simulink model "COSTEP_Exergy"  (R2024b)
settings: Solver=FixedStepAuto  StartTime=0.0  StopTime=25  FixedStep=1/3600  RelTol=1e-3
model workspace (MAT data in the model file):
  AD : Simulink.Parameter (value not decoded)
  AG : Simulink.Parameter (value not decoded)
  AH : Simulink.Parameter (value not decoded)
  AV : Simulink.Parameter (value not decoded)
  AVP : Simulink.Parameter (value not decoded)
  BCHL : Simulink.Parameter (value not decoded)
  BCHV : Simulink.Parameter (value not decoded)
  BD : Simulink.Parameter (value not decoded)
  BDIST : Simulink.Parameter (value not decoded)
  BG : Simulink.Parameter (value not decoded)
  BH : Simulink.Parameter (value not decoded)
  BVP : Simulink.Parameter (value not decoded)
  CD : Simulink.Parameter (value not decoded)
  CDIST : Simulink.Parameter (value not decoded)
  CG : Simulink.Parameter (value not decoded)
  CH : Simulink.Parameter (value not decoded)
  CVP : Simulink.Parameter (value not decoded)
  DDIST : Simulink.Parameter (value not decoded)
  DIST_CONST : Simulink.Parameter (value not decoded)
  ISV : Simulink.Parameter (value not decoded)
  TLAST : Simulink.Parameter (value not decoded)
  TNEXT : Simulink.Parameter (value not decoded)
  XMW : Simulink.Parameter (value not decoded)
  XNS : Simulink.Parameter (value not decoded)
  XNS2 : Simulink.Parameter (value not decoded)
  XNS3 : Simulink.Parameter (value not decoded)
  XNSADD : Simulink.Parameter (value not decoded)
  XNSE : Simulink.Parameter (value not decoded)
symbols that are objects in the model workspace (value not decoded): AD, AG, AH, AV, AVP, BD, BG, BH, BVP, CD, CG, CH, CVP, XMW, XNS, XNS2, XNS3, XNSE
undefined symbols (not defined in the file or in its folder): magnitude, msgbox, SETPT, XMEAS, XMV
libraries: mylib x403, dspindex x31
(part 8 of 13)

== system COSTEP_Exergy/Stripper/Holdup of Components in Stripper/Holsup of Liquid Components in Stripper ==
  YY(19:26) : Inport
  Bus Creator : BusCreator  Inputs=8
  Bus Selector : BusSelector  OutputSignals=YY(19),YY(20),YY(21),YY(22),YY(23),YY(24),YY(25),YY(26)
  UCLC(1) Holdup of Component A (Liquid) in Stripper lb-mol : Gain
  UCLC(2) Holdup of Component B (Liquid) in Stripper lb-mol : Gain
  UCLC(3) Holdup of Component C (Liquid) in Stripper lb-mol : Gain
  UCLC(4) Holdup of Component D (Liquid) in Stripper lb-mol : Gain
  UCLC(5) Holdup of Component E (Liquid) in Stripper lb-mol : Gain
  UCLC(6) Holdup of Component F (Liquid) in Stripper lb-mol : Gain
  UCLC(7) Holdup of Component G (Liquid) in Stripper lb-mol : Gain
  UCLC(8) Holdup of Component H (Liquid) in Stripper lb-mol : Gain
  UCLC : Outport  VectorParamsAs1DForOutWhenUnconnected=off
  wires:
  UCLC(8) Holdup of Component H (Liquid) in Stripper lb-mol/1 -> Bus Creator/8
  UCLC(2) Holdup of Component B (Liquid) in Stripper lb-mol/1 -> Bus Creator/2
  UCLC(1) Holdup of Component A (Liquid) in Stripper lb-mol/1 -> Bus Creator/1
  Bus Creator/1 -> UCLC/1
  UCLC(5) Holdup of Component E (Liquid) in Stripper lb-mol/1 -> Bus Creator/5
  UCLC(7) Holdup of Component G (Liquid) in Stripper lb-mol/1 -> Bus Creator/7
  UCLC(4) Holdup of Component D (Liquid) in Stripper lb-mol/1 -> Bus Creator/4
  UCLC(6) Holdup of Component F (Liquid) in Stripper lb-mol/1 -> Bus Creator/6
  UCLC(3) Holdup of Component C (Liquid) in Stripper lb-mol/1 -> Bus Creator/3
  YY(19:26)/1 -> Bus Selector/1
  Bus Selector/1 -> UCLC(1) Holdup of Component A (Liquid) in Stripper lb-mol/1  "<YY(19)>"
  Bus Selector/2 -> UCLC(2) Holdup of Component B (Liquid) in Stripper lb-mol/1  "<YY(20)>"
  Bus Selector/3 -> UCLC(3) Holdup of Component C (Liquid) in Stripper lb-mol/1  "<YY(21)>"
  Bus Selector/4 -> UCLC(4) Holdup of Component D (Liquid) in Stripper lb-mol/1  "<YY(22)>"
  Bus Selector/5 -> UCLC(5) Holdup of Component E (Liquid) in Stripper lb-mol/1  "<YY(23)>"
  Bus Selector/6 -> UCLC(6) Holdup of Component F (Liquid) in Stripper lb-mol/1  "<YY(24)>"
  Bus Selector/7 -> UCLC(7) Holdup of Component G (Liquid) in Stripper lb-mol/1  "<YY(25)>"
  Bus Selector/8 -> UCLC(8) Holdup of Component H (Liquid) in Stripper lb-mol/1  "<YY(26)>"

== system COSTEP_Exergy/Stripper/Holdup of Components in Stripper/Liquid Component Fraction in Stripper ==
  UTLC : Inport
  UCLC : Inport  Port=2
  Bus Selector : BusSelector  OutputSignals=signal1,signal2,signal3,signal4,signal5,signal6,signal7,signal8
  Mux : Mux  Inputs=8
  XLC(1) : Product  Inputs=*/
  XLC(2) : Product  Inputs=*/
  XLC(3) : Product  Inputs=*/
  XLC(4) : Product  Inputs=*/
  XLC(5) : Product  Inputs=*/
  XLC(6) : Product  Inputs=*/
  XLC(7) : Product  Inputs=*/
  XLC(8) : Product  Inputs=*/
  XLC : Outport  VectorParamsAs1DForOutWhenUnconnected=off
  wires:
  XLC(3)/1 -> Mux/3  "XLC(3)"
  Bus Selector/2 -> XLC(2)/1  "<signal2>"
  Bus Selector/7 -> XLC(7)/1  "<signal7>"
  XLC(5)/1 -> Mux/5  "XLC(5)"
  XLC(7)/1 -> Mux/7  "XLC(7)"
  Bus Selector/3 -> XLC(3)/1  "<signal3>"
  UTLC/1 -> XLC(8)/2, XLC(7)/2, XLC(6)/2, XLC(5)/2, XLC(4)/2, XLC(3)/2, XLC(2)/2, XLC(1)/2
  Bus Selector/6 -> XLC(6)/1  "<signal6>"
  Bus Selector/5 -> XLC(5)/1  "<signal5>"
  XLC(2)/1 -> Mux/2  "XLC(2)"
  XLC(6)/1 -> Mux/6  "XLC(6)"
  Bus Selector/4 -> XLC(4)/1  "<signal4>"
  XLC(1)/1 -> Mux/1  "XLC(1)"
  XLC(8)/1 -> Mux/8  "XLC(8)"
  UCLC/1 -> Bus Selector/1
  XLC(4)/1 -> Mux/4  "XLC(4)"
  Mux/1 -> XLC/1
  Bus Selector/1 -> XLC(1)/1  "<signal1>"
  Bus Selector/8 -> XLC(8)/1  "<signal8>"

== system COSTEP_Exergy/Stripper/Holdup of Components in Stripper/YP(19) ==
  FCM(1,12) : Inport
  FCM(1,13) : Inport  Port=2
  " " : Sum  Inputs=+-
  Constant : Constant  Value=19
  Initial state variable : mylib/Initial state variable
  Integration : mylib/Integration  SystemSampleTime=-1  VariantActivationTime=update diagram  AllowFlexibleInterface=on  Latency=0  AutoFrameSizeCalculation=off
  YY(19) : Outport  VectorParamsAs1DForOutWhenUnconnected=off
  wires:
  Initial state variable/1 -> Integration/2
  FCM(1,13)/1 -> " "/2
  FCM(1,12)/1 -> " "/1
  " "/1 -> Integration/1
  Integration/1 -> YY(19)/1
  Constant/1 -> Initial state variable/1

== system COSTEP_Exergy/Stripper/Holdup of Components in Stripper/YP(20) ==
  FCM(2,12) : Inport
  FCM(2,13) : Inport  Port=2
  " " : Sum  Inputs=+-
  Constant : Constant  Value=20
  Initial state variable : mylib/Initial state variable
  Integration : mylib/Integration  SystemSampleTime=-1  VariantActivationTime=update diagram  AllowFlexibleInterface=on  Latency=0  AutoFrameSizeCalculation=off
  YY(20) : Outport  VectorParamsAs1DForOutWhenUnconnected=off
  wires:
  Integration/1 -> YY(20)/1
  FCM(2,12)/1 -> " "/1
  FCM(2,13)/1 -> " "/2
  Initial state variable/1 -> Integration/2
  " "/1 -> Integration/1
  Constant/1 -> Initial state variable/1

== system COSTEP_Exergy/Stripper/Holdup of Components in Stripper/YP(21) ==
  FCM(3,12) : Inport
  FCM(3,13) : Inport  Port=2
  " " : Sum  Inputs=+-
  Constant : Constant  Value=21
  Initial state variable : mylib/Initial state variable
  Integration : mylib/Integration  SystemSampleTime=-1  VariantActivationTime=update diagram  AllowFlexibleInterface=on  Latency=0  AutoFrameSizeCalculation=off
  YY(21) : Outport  VectorParamsAs1DForOutWhenUnconnected=off
  wires:
  Integration/1 -> YY(21)/1
  FCM(3,12)/1 -> " "/1
  FCM(3,13)/1 -> " "/2
  " "/1 -> Integration/1
  Initial state variable/1 -> Integration/2
  Constant/1 -> Initial state variable/1

== system COSTEP_Exergy/Stripper/Holdup of Components in Stripper/YP(22) ==
  FCM(4,12) : Inport
  FCM(4,13) : Inport  Port=2
  " " : Sum  Inputs=+-
  Constant : Constant  Value=22
  Initial state variable : mylib/Initial state variable
  Integration : mylib/Integration  SystemSampleTime=-1  VariantActivationTime=update diagram  AllowFlexibleInterface=on  Latency=0  AutoFrameSizeCalculation=off
  "YY(22)  " : Outport  VectorParamsAs1DForOutWhenUnconnected=off
  wires:
  Integration/1 -> "YY(22)  "/1
  FCM(4,12)/1 -> " "/1
  FCM(4,13)/1 -> " "/2
  " "/1 -> Integration/1
  Initial state variable/1 -> Integration/2
  Constant/1 -> Initial state variable/1

== system COSTEP_Exergy/Stripper/Holdup of Components in Stripper/YP(23) ==
  FCM(5,12) : Inport
  FCM(5,13) : Inport  Port=2
  " " : Sum  Inputs=+-
  Constant : Constant  Value=23
  Initial state variable : mylib/Initial state variable
  Integration : mylib/Integration  SystemSampleTime=-1  VariantActivationTime=update diagram  AllowFlexibleInterface=on  Latency=0  AutoFrameSizeCalculation=off
  "YY(23)  " : Outport  VectorParamsAs1DForOutWhenUnconnected=off
  wires:
  Integration/1 -> "YY(23)  "/1
  FCM(5,12)/1 -> " "/1
  FCM(5,13)/1 -> " "/2
  " "/1 -> Integration/1
  Initial state variable/1 -> Integration/2
  Constant/1 -> Initial state variable/1

== system COSTEP_Exergy/Stripper/Holdup of Components in Stripper/YP(24) ==
  FCM(6,12) : Inport
  FCM(6,13) : Inport  Port=2
  " " : Sum  Inputs=+-
  Constant : Constant  Value=24
  Initial state variable : mylib/Initial state variable
  Integration : mylib/Integration  SystemSampleTime=-1  VariantActivationTime=update diagram  AllowFlexibleInterface=on  Latency=0  AutoFrameSizeCalculation=off
  "YY(24)  " : Outport  VectorParamsAs1DForOutWhenUnconnected=off
  wires:
  Integration/1 -> "YY(24)  "/1
  FCM(6,12)/1 -> " "/1
  FCM(6,13)/1 -> " "/2
  " "/1 -> Integration/1
  Initial state variable/1 -> Integration/2
  Constant/1 -> Initial state variable/1

== system COSTEP_Exergy/Stripper/Holdup of Components in Stripper/YP(25) ==
  FCM(7,12) : Inport
  FCM(7,13) : Inport  Port=2
  " " : Sum  Inputs=+-
  Constant : Constant  Value=25
  Initial state variable : mylib/Initial state variable
  Integration : mylib/Integration  SystemSampleTime=-1  VariantActivationTime=update diagram  AllowFlexibleInterface=on  Latency=0  AutoFrameSizeCalculation=off
  "YY(25)  " : Outport  VectorParamsAs1DForOutWhenUnconnected=off
  wires:
  Integration/1 -> "YY(25)  "/1
  FCM(7,12)/1 -> " "/1
  FCM(7,13)/1 -> " "/2
  " "/1 -> Integration/1
  Initial state variable/1 -> Integration/2
  Constant/1 -> Initial state variable/1

== system COSTEP_Exergy/Stripper/Holdup of Components in Stripper/YP(26) ==
  FCM(8,12) : Inport
  FCM(8,13) : Inport  Port=2
  " " : Sum  Inputs=+-
  Constant : Constant  Value=26
  Initial state variable : mylib/Initial state variable
  Integration : mylib/Integration  SystemSampleTime=-1  VariantActivationTime=update diagram  AllowFlexibleInterface=on  Latency=0  AutoFrameSizeCalculation=off
  "YY(26)   " : Outport  VectorParamsAs1DForOutWhenUnconnected=off
  wires:
  Integration/1 -> "YY(26)   "/1
  FCM(8,12)/1 -> " "/1
  FCM(8,13)/1 -> " "/2
  " "/1 -> Integration/1
  Initial state variable/1 -> Integration/2
  Constant/1 -> Initial state variable/1

== system COSTEP_Exergy/Stripper/PTC Pressure of Liquid zone in stripper mmHg/VPR Vapour Pressure mmHg ==
  TCR : Inport
  AVP(I) Antoine Coefficient A ln(mmHg) : Constant  Value=AVP
  Add : Sum
  Add1 : Sum
  BVP(I) Antoine Coefficient B ln(mmHg)·°C : Constant  Value=BVP
  CVP(I) Antoine Coefficient C °C : Constant  Value=CVP
  Divide : Product  Inputs=*/
  Math Function : Math  SignedPower=on
  VPR : Outport  VectorParamsAs1DForOutWhenUnconnected=off
  wires:
  BVP(I) Antoine Coefficient B ln(mmHg)·°C/1 -> Divide/1
  CVP(I) Antoine Coefficient C °C/1 -> Add/1
  AVP(I) Antoine Coefficient A ln(mmHg)/1 -> Add1/1
  Add/1 -> Divide/2
  Divide/1 -> Add1/2
  Add1/1 -> Math Function/1
  Math Function/1 -> VPR/1
  TCR/1 -> Add/2

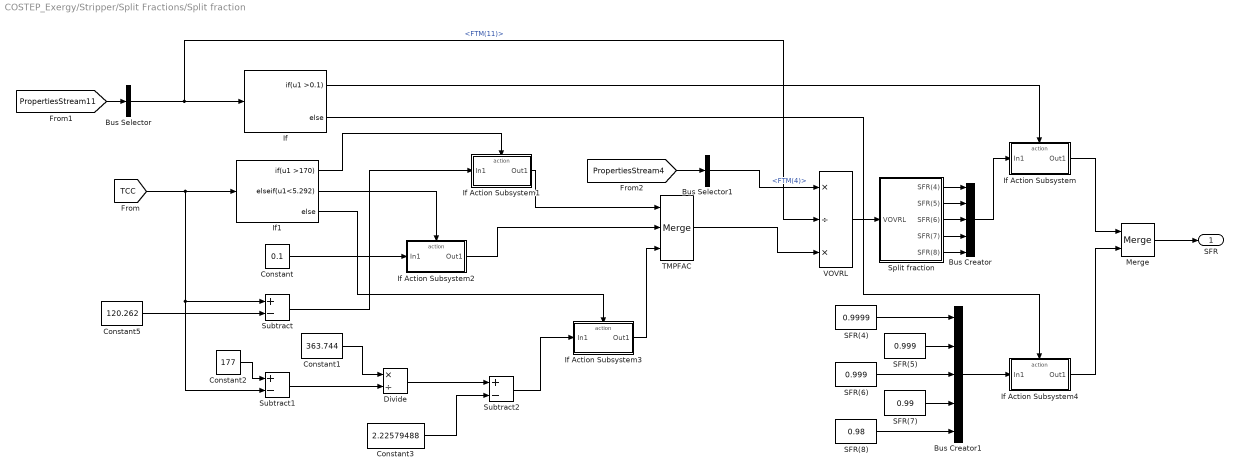
== system COSTEP_Exergy/Stripper/Split Fractions/Split fraction ==
  Bus Creator : BusCreator  Inputs=5
  Bus Creator1 : BusCreator  Inputs=5
  Bus Selector : BusSelector  OutputSignals=signal1.FTM(11)
  Bus Selector1 : BusSelector  OutputSignals=FTM(4)
  Constant : Constant  Value=0.1
  Constant1 : Constant  Value=363.744
  Constant2 : Constant  Value=177
  Constant3 : Constant  Value=2.22579488
  Constant5 : Constant  Value=120.262
  Divide : Product  Inputs=*/
  If : If  IfExpression=u1 >0.1
  If Action Subsystem : Subsystem  TreatAsAtomicUnit=on
  If Action Subsystem1 : Subsystem  TreatAsAtomicUnit=on
  If Action Subsystem2 : Subsystem  TreatAsAtomicUnit=on
  If Action Subsystem3 : Subsystem  TreatAsAtomicUnit=on
  If Action Subsystem4 : Subsystem  TreatAsAtomicUnit=on
  If1 : If  IfExpression=u1 >170  ElseIfExpressions=u1<5.292
  Merge : Merge
  SFR(4) : Constant  Value=0.9999
  SFR(5) : Constant  Value=0.999
  SFR(6) : Constant  Value=0.999
  SFR(7) : Constant  Value=0.99
  SFR(8) : Constant  Value=0.98
  Split fraction : Subsystem
  Subtract : Sum  Inputs=+-
  Subtract1 : Sum  Inputs=+-
  Subtract2 : Sum  Inputs=+-
  "TMPFAC  " : Merge  Inputs=3
  VOVRL : Product  Inputs=*/*
  SFR : Outport  VectorParamsAs1DForOutWhenUnconnected=off
  wires:
  If/1 -> If Action Subsystem/Action
  Bus Selector/1 -> VOVRL/2, If/1  "<FTM(11)>"
  [TCC] -> If1/1, Subtract1/2, Subtract/1
  Constant5/1 -> Subtract/2
  Constant2/1 -> Subtract1/1
  Subtract1/1 -> Divide/2
  Constant1/1 -> Divide/1
  Divide/1 -> Subtract2/1
  Constant3/1 -> Subtract2/2
  If Action Subsystem1/1(Out1) -> "TMPFAC  "/1
  If Action Subsystem2/1(Out1) -> "TMPFAC  "/2
  If1/1 -> If Action Subsystem1/Action
  Subtract/1 -> If Action Subsystem1/1(In1)
  If1/2 -> If Action Subsystem2/Action
  Constant/1 -> If Action Subsystem2/1(In1)
  Subtract2/1 -> If Action Subsystem3/1(In1)
  If1/3 -> If Action Subsystem3/Action
  If Action Subsystem3/1(Out1) -> "TMPFAC  "/3
  Bus Selector1/1 -> VOVRL/1  "<FTM(4)>"
  "TMPFAC  "/1 -> VOVRL/3
  VOVRL/1 -> Split fraction/1(VOVRL)
  If/2 -> If Action Subsystem4/Action
  Split fraction/1(SFR(4)) -> Bus Creator/1
  Split fraction/2(SFR(5)) -> Bus Creator/2
  Split fraction/3(SFR(6)) -> Bus Creator/3
  Split fraction/4(SFR(7)) -> Bus Creator/4
  Split fraction/5(SFR(8)) -> Bus Creator/5
  Bus Creator/1 -> If Action Subsystem/1(In1)
  Bus Creator1/1 -> If Action Subsystem4/1(In1)
  SFR(4)/1 -> Bus Creator1/1
  SFR(5)/1 -> Bus Creator1/2
  SFR(6)/1 -> Bus Creator1/3
  SFR(7)/1 -> Bus Creator1/4
  SFR(8)/1 -> Bus Creator1/5
  If Action Subsystem4/1(Out1) -> Merge/2
  If Action Subsystem/1(Out1) -> Merge/1
  Merge/1 -> SFR/1
  [PropertiesStream11] -> Bus Selector/1
  [PropertiesStream4] -> Bus Selector1/1

== system COSTEP_Exergy/Stripper/Stream 12/HST(12) Molar Enthalpy of Stream 12 MBtu//lb-mol ==
  ITY : Inport
  T : Inport  Port=2
  XST(I,I) : Inport  Port=3
  "Enthalpy of Stream " : mylib/Enthalpy of Stream   SystemSampleTime=-1  VariantActivationTime=update diagram  AllowFlexibleInterface=on  Latency=0  AutoFrameSizeCalculation=off
  "H " : Outport  VectorParamsAs1DForOutWhenUnconnected=off
  wires:
  ITY/1 -> "Enthalpy of Stream "/1
  T/1 -> "Enthalpy of Stream "/2
  XST(I,I)/1 -> "Enthalpy of Stream "/3
  "Enthalpy of Stream "/1 -> "H "/1

== system COSTEP_Exergy/Stripper/Stream 13/HST(13) Molar Enthalpy of Stream 13 MBtu//lb-mol ==
  ITY : Inport
  T : Inport  Port=2
  XST(I,I) : Inport  Port=3
  "Enthalpy of Stream " : mylib/Enthalpy of Stream   SystemSampleTime=-1  VariantActivationTime=update diagram  AllowFlexibleInterface=on  Latency=0  AutoFrameSizeCalculation=off
  "H " : Outport  VectorParamsAs1DForOutWhenUnconnected=off
  wires:
  ITY/1 -> "Enthalpy of Stream "/1
  T/1 -> "Enthalpy of Stream "/2
  XST(I,I)/1 -> "Enthalpy of Stream "/3
  "Enthalpy of Stream "/1 -> "H "/1

== system COSTEP_Exergy/Stripper/Stream 5/HST(5) Molar Enthalpy of Stream 5 MBtu//lb-mol ==
  ITY : Inport
  TST(5) : Inport  Port=2
  XST(I,5) : Inport  Port=3
  "Enthalpy of Stream " : mylib/Enthalpy of Stream   SystemSampleTime=-1  VariantActivationTime=update diagram  AllowFlexibleInterface=on  Latency=0  AutoFrameSizeCalculation=off
  "H " : Outport  PortDimensions=1  VectorParamsAs1DForOutWhenUnconnected=off
  wires:
  ITY/1 -> "Enthalpy of Stream "/1
  TST(5)/1 -> "Enthalpy of Stream "/2
  XST(I,5)/1 -> "Enthalpy of Stream "/3
  "Enthalpy of Stream "/1 -> "H "/1

== system COSTEP_Exergy/Stripper/Volume of Stripper/DLC Molar Density of Liquids in Stripper lb-mol//ft³     ==
  XLC : Inport
  TCC : Inport  Port=2
  "DLC Molar Density of Liquids in Stripper lb-mol/ft³ " : Subsystem
  "DLC " : Outport  VectorParamsAs1DForOutWhenUnconnected=off
  wires:
  "DLC Molar Density of Liquids in Stripper lb-mol/ft³ "/1("R ") -> "DLC "/1
  TCC/1 -> "DLC Molar Density of Liquids in Stripper lb-mol/ft³ "/2(T)
  XLC/1 -> "DLC Molar Density of Liquids in Stripper lb-mol/ft³ "/1(X)

== system COSTEP_Exergy/Subsystem1/Condenser cooling water/CCin ==
  Subsystem : Subsystem
  Subsystem1 : Subsystem
  Subsystem3 : Subsystem
  tag scope: BMCC1=global, QS1=global
  wires:
  Subsystem/1(Bphm J/s) -> [BMCC1]  "BphmCC1"
  Subsystem3/1(Bph) -> Subsystem/1(Bph)  "BphCC1"
  [TCWS] -> Subsystem1/1(T), Subsystem3/1(TC)
  [FWS] -> Subsystem1/2(F), Subsystem/2(FWS)
  Subsystem1/1(Q J/s) -> [QS1]

== system COSTEP_Exergy/Subsystem1/Condenser cooling water/CCout ==
  Subsystem : Subsystem
  Subsystem1 : Subsystem
  Subsystem3 : Subsystem
  tag scope: BMCC2=global, QS2=global
  wires:
  Subsystem/1(Bphm J/s) -> [BMCC2]  "BphmCC2"
  Subsystem3/1(Bph) -> Subsystem/1(Bph)  "BphCC2"
  [TWS] -> Subsystem1/1(T), Subsystem3/1(TC)
  [FWS] -> Subsystem1/2(F), Subsystem/2(FWS)
  Subsystem1/1(Q J/s) -> [QS2]

== system COSTEP_Exergy/Subsystem1/Reactor cooling water/RCin ==
  Subsystem : Subsystem
  Subsystem1 : Subsystem
  Subsystem3 : Subsystem
  tag scope: BMRC1=global, QR1=global
  wires:
  [TCWR] -> Subsystem1/1(T), Subsystem3/1(TC)
  Subsystem/1(Bphm J/s) -> [BMRC1]  "BphmRC1"
  Subsystem3/1(Bph) -> Subsystem/1(Bph)  "BphRC1"
  [FWR] -> Subsystem1/2(F), Subsystem/2(FWR)
  Subsystem1/1(Q J/s) -> [QR1]

== system COSTEP_Exergy/Subsystem1/Reactor cooling water/RCout ==
  Subsystem : Subsystem
  Subsystem1 : Subsystem
  Subsystem3 : Subsystem
  tag scope: BMRC2=global, QR2=global
  wires:
  Subsystem/1(Bphm J/s) -> [BMRC2]  "BphmRC2"
  Subsystem3/1(Bph) -> Subsystem/1(Bph)  "BphRC2"
  [TWR] -> Subsystem1/1(T), Subsystem3/1(TC)
  [FWR] -> Subsystem1/2(F), Subsystem/2(FWR)
  Subsystem1/1(Q J/s) -> [QR2]

== system COSTEP_Exergy/Control Mode/Braatz/ /CONTROL 1 ==
  XMEAS(2) : Inport
  SETPT(1) : Inport  Port=2
  P Control Velocity form : mylib/Braatz Control/P Control Velocity form  Kc=GAIN1  Ts=SI1  X_0=XMV1_0  H=HIGH1
  XMV(1) : Outport  VectorParamsAs1DForOutWhenUnconnected=off
  wires:
  SETPT(1)/1 -> P Control Velocity form/1
  P Control Velocity form/1 -> XMV(1)/1
  XMEAS(2)/1 -> P Control Velocity form/2

== system COSTEP_Exergy/Control Mode/Braatz/ /CONTROL 14 ==
  XMEAS(26) : Inport
  Constant : Constant  Value=SETPT14
  PI Control Setpoint Velocity form : Subsystem  mask{Kc=GAIN14, Ti=TAUI14, Ts=SI14, X_0=SETPT1, H=HIGH1, HS=HIGH14}
      mask prompts: Kc "Controller Gain - Kc"; Ti "Integral Time - Ti"; Ts "Sampling Interval - Ts"; X_0 "Initial Value"; H "High limit of measurment"; HS "High limit of setpoint"
      mask DialogControl DescGroupVar Prompt: Control Parameters
  SETPT(1) : Outport  VectorParamsAs1DForOutWhenUnconnected=off
  wires:
  Constant/1 -> PI Control Setpoint Velocity form/1(Setpoint)
  XMEAS(26)/1 -> PI Control Setpoint Velocity form/2(Measurement)
  PI Control Setpoint Velocity form/1(Output) -> SETPT(1)/1

== system COSTEP_Exergy/Control Mode/Braatz/ 1/CONTROL 15 ==
  XMEAS(27) : Inport
  Constant : Constant  Value=SETPT15
  PI Control Setpoint Velocity form : mylib/Braatz Control/PI Control Setpoint Velocity form  Kc=GAIN15  Ti=TAUI15  Ts=SI15  X_0=SETPT2  H=HIGH2  HS=HIGH15
  SETPT(2) : Outport  VectorParamsAs1DForOutWhenUnconnected=off
  wires:
  Constant/1 -> PI Control Setpoint Velocity form/1
  XMEAS(27)/1 -> PI Control Setpoint Velocity form/2
  PI Control Setpoint Velocity form/1 -> SETPT(2)/1

== system COSTEP_Exergy/Control Mode/Braatz/ 1/CONTROL 2 ==
  XMEAS(2) : Inport
  SETPT(2) : Inport  Port=2
  P Control Velocity form : mylib/Braatz Control/P Control Velocity form  Kc=GAIN2  Ts=SI2  X_0=XMV2_0  H=HIGH2
  XMV(2) : Outport  VectorParamsAs1DForOutWhenUnconnected=off
  wires:
  SETPT(2)/1 -> P Control Velocity form/1
  P Control Velocity form/1 -> XMV(2)/1
  XMEAS(2)/1 -> P Control Velocity form/2

== system COSTEP_Exergy/Control Mode/Braatz/ 10/CONTROL 19 ==
  XMEAS(30) : Inport
  Constant : Constant  Value=SETPT19
  PI Control Setpoint Velocity form : mylib/Braatz Control/PI Control Setpoint Velocity form  Kc=GAIN19  Ti=TAUI19  Ts=SI19  X_0=SETPT6  H=HIGH6  HS=HIGH19
  SETPT(6) : Outport  VectorParamsAs1DForOutWhenUnconnected=off
  wires:
  Constant/1 -> PI Control Setpoint Velocity form/1
  XMEAS(30)/1 -> PI Control Setpoint Velocity form/2
  PI Control Setpoint Velocity form/1 -> SETPT(6)/1

== system COSTEP_Exergy/Control Mode/Braatz/ 10/CONTROL 6 ==
  SETPT(6) : Inport
  XMEAS : Inport  Port=2
  Bus Selector : BusSelector  OutputSignals=signal3.XMEAS(10)
  P Control Velocity form : Subsystem  mask{Kc=GAIN6, Ts=SI6, X_0=XMV6_0, H=HIGH6}
      mask prompts: Kc "Controller Gain - Kc"; Ts "Sampling Interval - Ts"; X_0 "Initial Value"; H "High Limit of measurement"
      mask DialogControl DescGroupVar Prompt: Control Parameters
  XMV(6) : Outport  VectorParamsAs1DForOutWhenUnconnected=off
  wires:
  SETPT(6)/1 -> P Control Velocity form/1(Setpoint)
  P Control Velocity form/1(Output) -> XMV(6)/1
  Bus Selector/1 -> P Control Velocity form/2(Measurement)  "<XMEAS(10)>"
  XMEAS/1 -> P Control Velocity form/3(XMEAS), Bus Selector/1

== system COSTEP_Exergy/Control Mode/Braatz/ 2/CONTROL 13 ==
  XMEAS(23) : Inport
  Constant : Constant  Value=SETPT13
  PI Control Setpoint Velocity form : mylib/Braatz Control/PI Control Setpoint Velocity form  Kc=GAIN13  Ti=TAUI13  Ts=SI13  X_0=SETPT3  H=HIGH3  HS=HIGH13
  SETPT(3) : Outport  VectorParamsAs1DForOutWhenUnconnected=off
  wires:
  Constant/1 -> PI Control Setpoint Velocity form/1
  XMEAS(23)/1 -> PI Control Setpoint Velocity form/2
  PI Control Setpoint Velocity form/1 -> SETPT(3)/1

== system COSTEP_Exergy/Control Mode/Braatz/ 2/CONTROL 3 ==
  XMEAS(1) : Inport
  SETPT(3) : Inport  Port=2
  P Control Velocity form : mylib/Braatz Control/P Control Velocity form  Kc=GAIN3  Ts=SI3  X_0=XMV3_0  H=HIGH3
  XMV(3) : Outport
  wires:
  XMEAS(1)/1 -> P Control Velocity form/2
  P Control Velocity form/1 -> XMV(3)/1
  SETPT(3)/1 -> P Control Velocity form/1

== system COSTEP_Exergy/Control Mode/Braatz/ 3/CONTROL 17 ==
  XMEAS(8) : Inport
  Constant : Constant  Value=SETPT17
  PI Control Setpoint Velocity form : mylib/Braatz Control/PI Control Setpoint Velocity form  Kc=GAIN17  Ti=TAUI17  Ts=SI17  X_0=SETPT4  H=HIGH4  HS=HIGH17
  SETPT(4) : Outport  VectorParamsAs1DForOutWhenUnconnected=off
  wires:
  Constant/1 -> PI Control Setpoint Velocity form/1
  XMEAS(8)/1 -> PI Control Setpoint Velocity form/2
  PI Control Setpoint Velocity form/1 -> SETPT(4)/1

== system COSTEP_Exergy/Control Mode/Braatz/ 3/CONTROL 4 ==
  XMEAS(4) : Inport
  SETPT(4) : Inport  Port=2
  P Control Velocity form : mylib/Braatz Control/P Control Velocity form  Kc=GAIN4  Ts=SI4  X_0=XMV4_0  H=HIGH4
  XMV(4) : Outport  VectorParamsAs1DForOutWhenUnconnected=off
  wires:
  P Control Velocity form/1 -> XMV(4)/1
  XMEAS(4)/1 -> P Control Velocity form/2
  SETPT(4)/1 -> P Control Velocity form/1

== system COSTEP_Exergy/Control Mode/Braatz/ 4/CONTROL 5 ==
  XMEAS(5) : Inport
  Constant4 : Constant  Value=SETPT5
  PI Control Measurement Velocity form : mylib/Braatz Control/PI Control Measurement Velocity form  Kc=GAIN5  Ti=TAUI5  Ts=SI5  X_0=XMV5_0  H=HIGH5
  XMV(5) : Outport  VectorParamsAs1DForOutWhenUnconnected=off
  wires:
  XMEAS(5)/1 -> PI Control Measurement Velocity form/2
  PI Control Measurement Velocity form/1 -> XMV(5)/1
  Constant4/1 -> PI Control Measurement Velocity form/1

== system COSTEP_Exergy/Control Mode/Braatz/ 5/CONTROL 7 ==
  XMEAS(12) : Inport
  Constant4 : Constant  Value=SETPT7
  P Control Velocity form : mylib/Braatz Control/P Control Velocity form  Kc=GAIN7  Ts=SI7  X_0=XMV7_0  H=HIGH7
  XMV(7) : Outport  VectorParamsAs1DForOutWhenUnconnected=off
  wires:
  P Control Velocity form/1 -> XMV(7)/1
  Constant4/1 -> P Control Velocity form/1
  XMEAS(12)/1 -> P Control Velocity form/2

== system COSTEP_Exergy/Control Mode/Braatz/ 6/CONTROL 8 ==
  XMEAS(15) : Inport
  Constant4 : Constant  Value=SETPT8
  P Control Velocity form : mylib/Braatz Control/P Control Velocity form  Kc=GAIN8  Ts=SI8  X_0=XMV8_0  H=HIGH8
  XMV(8) : Outport  VectorParamsAs1DForOutWhenUnconnected=off
  wires:
  P Control Velocity form/1 -> XMV(8)/1
  Constant4/1 -> P Control Velocity form/1
  XMEAS(15)/1 -> P Control Velocity form/2

== system COSTEP_Exergy/Control Mode/Braatz/ 7/CONTROL 11 ==
  XMEAS(17) : Inport
  Constant4 : Constant  Value=SETPT11
  PI Control Measurement Velocity form : mylib/Braatz Control/PI Control Measurement Velocity form  Kc=GAIN11  Ti=TAUI11  Ts=SI11  X_0=XMV11_0  H=HIGH11
  XMV(11) : Outport  VectorParamsAs1DForOutWhenUnconnected=off
  wires:
  PI Control Measurement Velocity form/1 -> XMV(11)/1
  Constant4/1 -> PI Control Measurement Velocity form/1
  XMEAS(17)/1 -> PI Control Measurement Velocity form/2

== system COSTEP_Exergy/Control Mode/Braatz/ 8/CONTROL 10 ==
  XMEAS(21) : Inport
  SETPT(10) : Inport  Port=2
  PI Control Measurement Velocity form : mylib/Braatz Control/PI Control Measurement Velocity form  Kc=GAIN10  Ti=TAUI10  Ts=SI10  X_0=XMV10_0  H=HIGH10
  XMV(10) : Outport  VectorParamsAs1DForOutWhenUnconnected=off
  wires:
  PI Control Measurement Velocity form/1 -> XMV(10)/1
  SETPT(10)/1 -> PI Control Measurement Velocity form/1
  XMEAS(21)/1 -> PI Control Measurement Velocity form/2

== system COSTEP_Exergy/Control Mode/Braatz/ 8/CONTROL 18 ==
  XMEAS(9) : Inport
  Constant : Constant  Value=SETPT18
  PI Control Setpoint Velocity form : mylib/Braatz Control/PI Control Setpoint Velocity form  Kc=GAIN18  Ti=TAUI18  Ts=SI18  X_0=SETPT10  H=HIGH10  HS=HIGH18
  SETPT(10) : Outport  VectorParamsAs1DForOutWhenUnconnected=off
  wires:
  Constant/1 -> PI Control Setpoint Velocity form/1
  XMEAS(9)/1 -> PI Control Setpoint Velocity form/2
  PI Control Setpoint Velocity form/1 -> SETPT(10)/1

== system COSTEP_Exergy/Control Mode/Braatz/ 9/CONTROL 16 ==
  XMEAS(18) : Inport
  SETPT(16) : Inport  Port=2
  PI Control Setpoint Velocity form : mylib/Braatz Control/PI Control Setpoint Velocity form  Kc=GAIN16  Ti=TAUI16  Ts=SI16  X_0=SETPT9  H=HIGH9  HS=HIGH16
  SETPT(9) : Outport  VectorParamsAs1DForOutWhenUnconnected=off
  wires:
  SETPT(16)/1 -> PI Control Setpoint Velocity form/1
  XMEAS(18)/1 -> PI Control Setpoint Velocity form/2
  PI Control Setpoint Velocity form/1 -> SETPT(9)/1

== system COSTEP_Exergy/Control Mode/Braatz/ 9/CONTROL 20 ==
  XMEAS(38) : Inport
  Constant : Constant  Value=SETPT20
  PI Control Setpoint Velocity form : mylib/Braatz Control/PI Control Setpoint Velocity form  Kc=GAIN20  Ti=TAUI20  Ts=SI20  X_0=SETPT16  H=HIGH16  HS=HIGH20
  SETPT(16) : Outport  VectorParamsAs1DForOutWhenUnconnected=off
  wires:
  Constant/1 -> PI Control Setpoint Velocity form/1
  XMEAS(38)/1 -> PI Control Setpoint Velocity form/2
  PI Control Setpoint Velocity form/1 -> SETPT(16)/1

== system COSTEP_Exergy/Control Mode/Braatz/ 9/CONTROL 9 ==
  XMEAS(19) : Inport
  SETPT(9) : Inport  Port=2
  P Control Velocity form : mylib/Braatz Control/P Control Velocity form  Kc=GAIN9  Ts=SI9  X_0=XMV9_0  H=HIGH9
  XMV(9) : Outport  VectorParamsAs1DForOutWhenUnconnected=off
  wires:
  SETPT(9)/1 -> P Control Velocity form/1
  P Control Velocity form/1 -> XMV(9)/1
  XMEAS(19)/1 -> P Control Velocity form/2

== system COSTEP_Exergy/Mixing Zone/Stream 6/Subsystem/If Action Subsystem ==
  In1 : Inport
  Action Port : ActionPort  ActionPortLabel=if(u1 < 0)
  Out1 : Outport  VectorParamsAs1DForOutWhenUnconnected=off
  wires:
  In1/1 -> Out1/1

== system COSTEP_Exergy/Mixing Zone/Stream 6/Subsystem/If Action Subsystem1 ==
  In1 : Inport
  Action Port : ActionPort  ActionPortLabel=else
  Out1 : Outport  VectorParamsAs1DForOutWhenUnconnected=off
  wires:
  In1/1 -> Out1/1

== system COSTEP_Exergy/Process Measurements/Feed Streams/D Feed/XMWS(1) Molecular weight of Stream 1 lb//lb-mol ==
  XST(I,1) : Inport
  Product : Product
  Sum of Elements : Sum  Inputs=+
  "XMW(I) Molecular weight of components lb/lb-mol " : Constant  Value=XMW
  XMWS(1) : Outport  VectorParamsAs1DForOutWhenUnconnected=off
  wires:
  Sum of Elements/1 -> XMWS(1)/1
  Product/1 -> Sum of Elements/1
  XST(I,1)/1 -> Product/1
  "XMW(I) Molecular weight of components lb/lb-mol "/1 -> Product/2

== system COSTEP_Exergy/Process Measurements/Feed Streams/E Feed/XMWS(2) Molecular weight of Stream 2 lb//lb-mol ==
  XST(I,2) : Inport
  Product : Product
  Sum of Elements : Sum  Inputs=+
  "XMW(I) Molecular weight of components lb/lb-mol " : Constant  Value=XMW
  XMWS(2) : Outport  VectorParamsAs1DForOutWhenUnconnected=off
  wires:
  Sum of Elements/1 -> XMWS(2)/1
  Product/1 -> Sum of Elements/1
  XST(I,2)/1 -> Product/1
  "XMW(I) Molecular weight of components lb/lb-mol "/1 -> Product/2

== system COSTEP_Exergy/Process Measurements/Product analysis/Subsystem/Subsystem ==
  XST : Inport
  Constant : Constant  Value=100
  Multiport Selector : dspindex/Multiport Selector  rowsOrCols=Rows  idxCellArray={4,5,6,7,8}  idxErrMode=Clip Index
  XCMP(37) : Product
  XCMP(38) : Product
  XCMP(39) : Product
  XCMP(40) : Product
  XCMP(41) : Product
  "XCMP(37) " : Outport  VectorParamsAs1DForOutWhenUnconnected=off
  "XCMP(38) " : Outport  Port=2  VectorParamsAs1DForOutWhenUnconnected=off
  "XCMP(39) " : Outport  Port=3  VectorParamsAs1DForOutWhenUnconnected=off
  "XCMP(40) " : Outport  Port=4  VectorParamsAs1DForOutWhenUnconnected=off
  "XCMP(41) " : Outport  Port=5  VectorParamsAs1DForOutWhenUnconnected=off
  wires:
  Constant/1 -> XCMP(38)/2, XCMP(40)/2, XCMP(41)/2, XCMP(39)/2, XCMP(37)/2
  Multiport Selector/1 -> XCMP(37)/1
  XCMP(37)/1 -> "XCMP(37) "/1  "XCMP(37)"
  Multiport Selector/5 -> XCMP(41)/1
  XCMP(39)/1 -> "XCMP(39) "/1  "XCMP(39)"
  XST/1 -> Multiport Selector/1
  Multiport Selector/4 -> XCMP(40)/1
  Multiport Selector/2 -> XCMP(38)/1
  Multiport Selector/3 -> XCMP(39)/1
  XCMP(38)/1 -> "XCMP(38) "/1  "XCMP(38)"
  XCMP(41)/1 -> "XCMP(41) "/1  "XCMP(41)"
  XCMP(40)/1 -> "XCMP(40) "/1  "XCMP(40)"

== system COSTEP_Exergy/Process Measurements/Purge gas analysis/Subsystem/Subsystem ==
  XST : Inport
  Constant : Constant  Value=100
  Multiport Selector : dspindex/Multiport Selector  rowsOrCols=Rows  idxCellArray={ 1,2,3,4,5,6,7,8}  idxErrMode=Clip Index
  XCMP(29) : Product
  XCMP(30) : Product
  XCMP(31) : Product
  XCMP(32) : Product
  XCMP(33) : Product
  XCMP(34) : Product
  XCMP(35) : Product
  XCMP(36) : Product
  "XCMP(29) " : Outport  VectorParamsAs1DForOutWhenUnconnected=off
  "XCMP(30) " : Outport  Port=2  VectorParamsAs1DForOutWhenUnconnected=off
  "XCMP(31) " : Outport  Port=3  VectorParamsAs1DForOutWhenUnconnected=off
  "XCMP(32) " : Outport  Port=4  VectorParamsAs1DForOutWhenUnconnected=off
  "XCMP(33) " : Outport  Port=5  VectorParamsAs1DForOutWhenUnconnected=off
  "XCMP(34) " : Outport  Port=6  VectorParamsAs1DForOutWhenUnconnected=off
  "XCMP(35) " : Outport  Port=7  VectorParamsAs1DForOutWhenUnconnected=off
  "XCMP(36) " : Outport  Port=8  VectorParamsAs1DForOutWhenUnconnected=off
  wires:
  XCMP(32)/1 -> "XCMP(32) "/1  "XCMP(32)"
  Multiport Selector/6 -> XCMP(34)/1
  Multiport Selector/8 -> XCMP(36)/1
  XCMP(29)/1 -> "XCMP(29) "/1  "XCMP(29)"
  Multiport Selector/5 -> XCMP(33)/1
  Multiport Selector/7 -> XCMP(35)/1
  XCMP(30)/1 -> "XCMP(30) "/1  "XCMP(30)"
  Multiport Selector/1 -> XCMP(29)/1
  Multiport Selector/3 -> XCMP(31)/1
  Constant/1 -> XCMP(32)/2, XCMP(36)/2, XCMP(35)/2, XCMP(34)/2, XCMP(33)/2, XCMP(31)/2, XCMP(30)/2, XCMP(29)/2
  XCMP(33)/1 -> "XCMP(33) "/1  "XCMP(33)"
  Multiport Selector/4 -> XCMP(32)/1
  XST/1 -> Multiport Selector/1
  Multiport Selector/2 -> XCMP(30)/1
  XCMP(31)/1 -> "XCMP(31) "/1  "XCMP(31)"
  XCMP(35)/1 -> "XCMP(35) "/1  "XCMP(35)"
  XCMP(36)/1 -> "XCMP(36) "/1  "XCMP(36)"
  XCMP(34)/1 -> "XCMP(34) "/1  "XCMP(34)"

== system COSTEP_Exergy/Process Measurements/Reactor feed analysis/Subsystem/Subsystem ==
  XST : Inport
  Constant : Constant  Value=100
  Multiport Selector : dspindex/Multiport Selector  rowsOrCols=Rows  idxCellArray={ 1,2,3,4,5,6,}  idxErrMode=Clip Index
  XCMP(23) : Product
  XCMP(24) : Product
  XCMP(25) : Product
  XCMP(26) : Product
  XCMP(27) : Product
  XCMP(28) : Product
  XCMP(23)1 : Outport  VectorParamsAs1DForOutWhenUnconnected=off
  XCMP(24)1 : Outport  Port=2  VectorParamsAs1DForOutWhenUnconnected=off
  XCMP(25)1 : Outport  Port=3  VectorParamsAs1DForOutWhenUnconnected=off
  XCMP(26)1 : Outport  Port=4  VectorParamsAs1DForOutWhenUnconnected=off
  XCMP(27)1 : Outport  Port=5  VectorParamsAs1DForOutWhenUnconnected=off
  XCMP(28)1 : Outport  Port=6  VectorParamsAs1DForOutWhenUnconnected=off
  wires:
  Multiport Selector/1 -> XCMP(23)/1  "XST(1;7)"
  Multiport Selector/4 -> XCMP(26)/1  "XST(4;7)"
  Constant/1 -> XCMP(26)/2, XCMP(28)/2, XCMP(27)/2, XCMP(25)/2, XCMP(24)/2, XCMP(23)/2
  Multiport Selector/2 -> XCMP(24)/1  "XST(2;7)"
  XST/1 -> Multiport Selector/1
  Multiport Selector/6 -> XCMP(28)/1  "XST(6:7)"
  Multiport Selector/3 -> XCMP(25)/1  "XST(3;7)"
  XCMP(23)/1 -> XCMP(23)1/1  "XCMP(23)"
  Multiport Selector/5 -> XCMP(27)/1  "XST(5;7)"
  XCMP(25)/1 -> XCMP(25)1/1  "XCMP(25)"
  XCMP(26)/1 -> XCMP(26)1/1  "XCMP(26)"
  XCMP(24)/1 -> XCMP(24)1/1  "XCMP(24)"
  XCMP(27)/1 -> XCMP(27)1/1  "XCMP(27)"
  XCMP(28)/1 -> XCMP(28)1/1  "XCMP(28)"

== system COSTEP_Exergy/Random number generator/Stream Measurements SMEAS Gas analysis1/Gas Analysis Delay/Subsystem ==
  In1 : Inport
  In2 : Inport  Port=2
  If : If  NumInputs=2  IfExpression=u1 == u2
  If Action Subsystem : Subsystem  TreatAsAtomicUnit=on
  If Action Subsystem1 : Subsystem  TreatAsAtomicUnit=on
  Rounding Function : Rounding  Operator=round
  Out1 : Outport  VectorParamsAs1DForOutWhenUnconnected=off
  Out2 : Outport  Port=2  VectorParamsAs1DForOutWhenUnconnected=off
  wires:
  Rounding Function/1 -> If/1, If Action Subsystem1/1(In1)
  In2/1 -> If/2
  If Action Subsystem/1(Out1) -> Out1/1
  If Action Subsystem1/1(Out1) -> Out2/1
  In1/1 -> Rounding Function/1
  If/1 -> If Action Subsystem/Action
  If/2 -> If Action Subsystem1/Action

== system COSTEP_Exergy/Random number generator/Stream Measurements SMEAS Gas analysis1/If Action Subsystem3/Subsystem ==
  G : Inport
  Bus Creator2 : BusCreator  Inputs=9
  Stream 1 : Subsystem
  Stream 13 : Subsystem
  Stream 2 : Subsystem
  Stream 3 : Subsystem
  Stream 4 : Subsystem
  Stream 5 : Subsystem
  Stream 6 : Subsystem
  Stream 8 : Subsystem
  Stream 9 : Subsystem
  XMNSE2 : Outport  VectorParamsAs1DForOutWhenUnconnected=off
  G_NEW : Outport  Port=2  VectorParamsAs1DForOutWhenUnconnected=off
  wires:
  Bus Creator2/1 -> XMNSE2/1
  G/1 -> Stream 1/1(G)
  Stream 1/1(Stream 1) -> Bus Creator2/1
  Stream 1/2(G_NEW) -> Stream 2/1(G)
  Stream 2/1(Stream 2) -> Bus Creator2/2
  Stream 2/2(G_NEW) -> Stream 3/1(G)
  Stream 3/1(Stream 3) -> Bus Creator2/3
  Stream 3/2(G_NEW) -> Stream 4/1(G)
  Stream 4/1(Stream 4) -> Bus Creator2/4
  Stream 4/2(G_NEW) -> Stream 5/1(G)
  Stream 5/1(Stream 5) -> Bus Creator2/5
  Stream 5/2(G_NEW) -> Stream 6/1(G)
  Stream 6/1(Stream 6) -> Bus Creator2/6
  Stream 6/2(G_NEW) -> Stream 8/1(G)
  Stream 8/1(Stream 8) -> Bus Creator2/7
  Stream 8/2(G_NEW) -> Stream 9/1(G)
  Stream 9/1(Stream 9) -> Bus Creator2/8
  Stream 9/2(G_NEW) -> Stream 13/1(G)
  Stream 13/2(G_NEW) -> G_NEW/1
  Stream 13/1(Stream 13) -> Bus Creator2/9

== system COSTEP_Exergy/Random number generator/Stream Measurements SMEAS Gas analysis1/Subsystem/If Action Subsystem ==
  In1 : Inport
  Action Port : ActionPort  ActionPortLabel=if(u1 == 0)
  Out1 : Outport  VectorParamsAs1DForOutWhenUnconnected=off
  wires:
  In1/1 -> Out1/1

== system COSTEP_Exergy/Random number generator/Stream Measurements SMEAS Gas analysis1/Subsystem/If Action Subsystem1 ==
  In1 : Inport
  Action Port : ActionPort  ActionPortLabel=else
  Out1 : Outport  VectorParamsAs1DForOutWhenUnconnected=off
  wires:
  In1/1 -> Out1/1

== system COSTEP_Exergy/Random number generator/Stream Measurements SMEAS Product analysis1/Gas Analysis Delay/Subsystem ==
  In1 : Inport
  In2 : Inport  Port=2
  If : If  NumInputs=2  IfExpression=u1 == u2
  If Action Subsystem : Subsystem  TreatAsAtomicUnit=on
  If Action Subsystem1 : Subsystem  TreatAsAtomicUnit=on
  Rounding Function : Rounding  Operator=round
  Out1 : Outport  VectorParamsAs1DForOutWhenUnconnected=off
  Out2 : Outport  Port=2  VectorParamsAs1DForOutWhenUnconnected=off
  wires:
  Rounding Function/1 -> If/1, If Action Subsystem1/1(In1)
  In2/1 -> If/2
  If Action Subsystem/1(Out1) -> Out1/1
  If Action Subsystem1/1(Out1) -> Out2/1
  In1/1 -> Rounding Function/1
  If/1 -> If Action Subsystem/Action
  If/2 -> If Action Subsystem1/Action

== system COSTEP_Exergy/Random number generator/Stream Measurements SMEAS Product analysis1/If Action Subsystem3/Subsystem ==
  G : Inport
  Bus Creator : BusCreator  Inputs=2
  Subsystem1 : Subsystem
  Subsystem2 : Subsystem
  XMNSE3 : Outport  VectorParamsAs1DForOutWhenUnconnected=off
  G_NEW : Outport  Port=2  VectorParamsAs1DForOutWhenUnconnected=off
  wires:
  G/1 -> Subsystem1/1(G)
  Subsystem1/1(Stream 11) -> Bus Creator/1
  Bus Creator/1 -> XMNSE3/1
  Subsystem1/2(G_NEW) -> Subsystem2/1(G)
  Subsystem2/1(Stream 13) -> Bus Creator/2
  Subsystem2/2(G_NEW) -> G_NEW/1

== system COSTEP_Exergy/Random number generator/Stream Measurements SMEAS Product analysis1/Subsystem/If Action Subsystem ==
  In1 : Inport
  Action Port : ActionPort  ActionPortLabel=if(u1 == 0)
  Out1 : Outport  VectorParamsAs1DForOutWhenUnconnected=off
  wires:
  In1/1 -> Out1/1

== system COSTEP_Exergy/Random number generator/Stream Measurements SMEAS Product analysis1/Subsystem/If Action Subsystem1 ==
  In1 : Inport
  Action Port : ActionPort  ActionPortLabel=else
  Out1 : Outport  VectorParamsAs1DForOutWhenUnconnected=off
  wires:
  In1/1 -> Out1/1

== system COSTEP_Exergy/Reactor/Reaction Rates/Component reaction rate lb-mol//h/Subsystem ==
  RR : Inport
  " " : Sum  Inputs=---
  Bus Selector : BusSelector  OutputSignals=RR(1),RR(2),RR(3)
  CRXR(1) : Outport  VectorParamsAs1DForOutWhenUnconnected=off
  wires:
  " "/1 -> CRXR(1)/1  "CRXR(1)"
  Bus Selector/2 -> " "/2  "<RR(2)>"
  Bus Selector/3 -> " "/3  "<RR(3)>"
  RR/1 -> Bus Selector/1
  Bus Selector/1 -> " "/1  "<RR(1)>"

== system COSTEP_Exergy/Reactor/Reaction Rates/Component reaction rate lb-mol//h/Subsystem1 ==
  RR : Inport
  " " : Sum  Inputs=--
  Bus Selector : BusSelector  OutputSignals=RR(1),RR(2)
  CRXR(3) : Outport  VectorParamsAs1DForOutWhenUnconnected=off
  wires:
  " "/1 -> CRXR(3)/1  "CRXR(3)"
  RR/1 -> Bus Selector/1
  Bus Selector/1 -> " "/1  "<RR(1)>"
  Bus Selector/2 -> " "/2  "<RR(2)>"

== system COSTEP_Exergy/Reactor/Reaction Rates/Component reaction rate lb-mol//h/Subsystem2 ==
  RR : Inport
  " " : Sum  Inputs=--
  Bus Selector : BusSelector  OutputSignals=RR(1),RR(4)
  Gain : Gain  Gain=1.5
  CRXR(4) : Outport  VectorParamsAs1DForOutWhenUnconnected=off
  wires:
  Gain/1 -> " "/2
  Bus Selector/1 -> " "/1  "<RR(1)>"
  " "/1 -> CRXR(4)/1  "CRXR(4)"
  RR/1 -> Bus Selector/1
  Bus Selector/2 -> Gain/1  "<RR(4)>"

== system COSTEP_Exergy/Reactor/Reaction Rates/Component reaction rate lb-mol//h/Subsystem3 ==
  RR : Inport
  " " : Sum  Inputs=--
  Bus Selector : BusSelector  OutputSignals=RR(2),RR(3)
  CRXR(5) : Outport  VectorParamsAs1DForOutWhenUnconnected=off
  wires:
  " "/1 -> CRXR(5)/1  "CRXR(5)"
  RR/1 -> Bus Selector/1
  Bus Selector/1 -> " "/1  "<RR(2)>"
  Bus Selector/2 -> " "/2  "<RR(3)>"

== system COSTEP_Exergy/Reactor/Reaction Rates/Component reaction rate lb-mol//h/Subsystem4 ==
  RR : Inport
  " " : Sum
  Bus Selector : BusSelector  OutputSignals=RR(3),RR(4)
  CRXR(6) : Outport  VectorParamsAs1DForOutWhenUnconnected=off
  wires:
  " "/1 -> CRXR(6)/1  "CRXR(6)"
  RR/1 -> Bus Selector/1
  Bus Selector/2 -> " "/2  "<RR(4)>"
  Bus Selector/1 -> " "/1  "<RR(3)>"

== system COSTEP_Exergy/Reactor/Reaction Rates/Component reaction rate lb-mol//h/Subsystem5 ==
  RR : Inport
  Bus Selector : BusSelector  OutputSignals=RR(1)
  Gain : Gain
  CRXR(7) : Outport  VectorParamsAs1DForOutWhenUnconnected=off
  wires:
  Bus Selector/1 -> Gain/1  "<RR(1)>"
  RR/1 -> Bus Selector/1
  Gain/1 -> CRXR(7)/1  "CRXR(7)"

== system COSTEP_Exergy/Reactor/Reaction Rates/Component reaction rate lb-mol//h/Subsystem6 ==
  RR : Inport
  " " : Gain
  Bus Selector : BusSelector  OutputSignals=RR(2)
  CRXR(8) : Outport  VectorParamsAs1DForOutWhenUnconnected=off
  wires:
  " "/1 -> CRXR(8)/1  "CRXR(8)"
  RR/1 -> Bus Selector/1
  Bus Selector/1 -> " "/1  "<RR(2)>"

== system COSTEP_Exergy/Reactor/Reaction Rates/Reaction rates lb-mol//h/ Reaction rate of reaction 4 lb-mol//ft3·h     ==
  PPR : Inport
  TKR : Inport  Port=2
  Activation energy cal/mol : Constant  Value=60000
  Bus Selector : BusSelector  OutputSignals=PPR(1),PPR(4)
  Divide : Product  Inputs=*//
  Divide1 : Product  Inputs=3
  Gain : Gain  Gain=0.767488334
  Math Function2 : Math  SignedPower=on
  Preexponential factor lb-mol/ft3·h·mmHg : Constant  Value=53.4060443
  Subtract : Sum  Inputs=+-
  Universal gas constant cal/mol·K : Constant  Value=1.987
  RR(4) : Outport  VectorParamsAs1DForOutWhenUnconnected=off
  wires:
  Divide/1 -> Subtract/2
  Universal gas constant cal/mol·K/1 -> Divide/2
  Preexponential factor lb-mol/ft3·h·mmHg/1 -> Subtract/1
  Activation energy cal/mol/1 -> Divide/1
  TKR/1 -> Divide/3
  Subtract/1 -> Math Function2/1
  Divide1/1 -> RR(4)/1
  Bus Selector/2 -> Divide1/3  "<PPR(4)>"
  Gain/1 -> Divide1/1
  Math Function2/1 -> Gain/1
  PPR/1 -> Bus Selector/1
  Bus Selector/1 -> Divide1/2  "<PPR(1)>"

== system COSTEP_Exergy/Reactor/Reaction Rates/Reaction rates lb-mol//h/Reaction rate of reaction 1 lb-mol//ft3·h ==
  PPR : Inport
  TKR : Inport  Port=2
  " " : Constant  Value=0
  Abs : Abs  SaturateOnIntegerOverflow=off
  Bus Selector : BusSelector  OutputSignals=PPR(1),PPR(3)
  If : If  NumInputs=2  IfExpression=u1>0 & u2>0
  If Action Subsystem : Subsystem  TreatAsAtomicUnit=on
  If Action Subsystem2 : Subsystem  TreatAsAtomicUnit=on
  Merge1 : Merge
  "RR(1) Reaction rate of 1st reaction lb-mol/ft3·h " : Subsystem
  RR(1) : Outport  VectorParamsAs1DForOutWhenUnconnected=off
  wires:
  "RR(1) Reaction rate of 1st reaction lb-mol/ft3·h "/1(RR(1)) -> If Action Subsystem/1(In1)
  If/1 -> If Action Subsystem/Action
  " "/1 -> If Action Subsystem2/1(In1)
  If/2 -> If Action Subsystem2/Action
  Merge1/1 -> Abs/1
  If Action Subsystem/1(Out1) -> Merge1/1
  If Action Subsystem2/1(Out1) -> Merge1/2
  TKR/1 -> "RR(1) Reaction rate of 1st reaction lb-mol/ft3·h "/2(TKR)
  Abs/1 -> RR(1)/1
  PPR/1 -> "RR(1) Reaction rate of 1st reaction lb-mol/ft3·h "/1(PPR), Bus Selector/1
  Bus Selector/1 -> If/1  "<PPR(1)>"
  Bus Selector/2 -> If/2  "<PPR(3)>"

== system COSTEP_Exergy/Reactor/Reaction Rates/Reaction rates lb-mol//h/Reaction rate of reaction 2 lb-mol//ft3·h ==
  PPR : Inport
  TKR : Inport  Port=2
  " " : Constant  Value=0
  Abs : Abs  SaturateOnIntegerOverflow=off
  Bus Selector : BusSelector  OutputSignals=PPR(1),PPR(3)
  If : If  NumInputs=2  IfExpression=u1>0 & u2>0
  If Action Subsystem : Subsystem  TreatAsAtomicUnit=on
  If Action Subsystem2 : Subsystem  TreatAsAtomicUnit=on
  Merge1 : Merge
  "RR(2) Reaction rate of 2nd reaction lb-mol/ft3·h " : Subsystem
  RR(2) : Outport  VectorParamsAs1DForOutWhenUnconnected=off
  wires:
  If/1 -> If Action Subsystem/Action
  If/2 -> If Action Subsystem2/Action
  "RR(2) Reaction rate of 2nd reaction lb-mol/ft3·h "/1(RR(2)) -> If Action Subsystem/1(In1)
  " "/1 -> If Action Subsystem2/1(In1)
  If Action Subsystem2/1(Out1) -> Merge1/2
  TKR/1 -> "RR(2) Reaction rate of 2nd reaction lb-mol/ft3·h "/2(TKR)
  If Action Subsystem/1(Out1) -> Merge1/1
  Merge1/1 -> Abs/1
  Abs/1 -> RR(2)/1
  PPR/1 -> "RR(2) Reaction rate of 2nd reaction lb-mol/ft3·h "/1(PPR), Bus Selector/1
  Bus Selector/1 -> If/1  "<PPR(1)>"
  Bus Selector/2 -> If/2  "<PPR(3)>"

== system COSTEP_Exergy/Reactor/Reaction Rates/Reaction rates lb-mol//h/Reaction rate of reaction 3 lb-mol//ft3·h   ==
  PPR : Inport
  TKR : Inport  Port=2
  Activation energy cal/mol : Constant  Value=60000
  Bus Selector : BusSelector  OutputSignals=PPR(1),PPR(5)
  Divide : Product  Inputs=*//
  Divide1 : Product  Inputs=3
  Math Function2 : Math  SignedPower=on
  Preexponential factor lb-mol/ft3·h·mmHg : Constant  Value=53.4060443
  Subtract : Sum  Inputs=+-
  Universal gas constant cal/mol·K : Constant  Value=1.987
  RR(3) : Outport  VectorParamsAs1DForOutWhenUnconnected=off
  wires:
  Divide/1 -> Subtract/2
  Universal gas constant cal/mol·K/1 -> Divide/2
  Preexponential factor lb-mol/ft3·h·mmHg/1 -> Subtract/1
  Activation energy cal/mol/1 -> Divide/1
  TKR/1 -> Divide/3
  Subtract/1 -> Math Function2/1
  Bus Selector/2 -> Divide1/3  "<PPR(5)>"
  Divide1/1 -> RR(3)/1
  Math Function2/1 -> Divide1/1
  PPR/1 -> Bus Selector/1
  Bus Selector/1 -> Divide1/2  "<PPR(1)>"

== system COSTEP_Exergy/Reactor/Reactor Heat exchanger/Position of Valve 12 %/Control valve ==
  XMV(12) : Inport
  Saturation : Saturate  UpperLimit=100  LowerLimit=0
  VCV(12) : Outport  PortDimensions=1  VectorParamsAs1DForOutWhenUnconnected=off
  wires:
  Saturation/1 -> VCV(12)/1
  XMV(12)/1 -> Saturation/1

== system COSTEP_Exergy/Reactor/Reactor Heat exchanger/Reactor Heat exchanger/AGSP Agitation speed ==
  VPOS(12) : Inport
  " " : Product  Inputs=*/
  Add : Sum
  Constant1 : Constant  Value=150
  Constant2 : Constant  Value=100
  AGSP : Outport  VectorParamsAs1DForOutWhenUnconnected=off
  wires:
  Constant2/1 -> " "/2
  " "/1 -> AGSP/1
  VPOS(12)/1 -> Add/1
  Constant1/1 -> Add/2
  Add/1 -> " "/1

== system COSTEP_Exergy/Reactor/Reactor Heat exchanger/Reactor Heat exchanger/Cooling water outlet temperature ==
  FWR : Inport
  QUR : Inport  Port=2  PortDimensions=1
  Constant : Constant  Value=37
  Constant1 : Constant  Value=1e6
  Constant2 : Constant  Value=1.8
  Constant6 : Constant  Value=500.53
  Divide : Product  Inputs=*/
  Divide1 : Product
  Divide2 : Product  Inputs=*/
  HWR : Constant  Value=7060
  Initial state variable : mylib/Initial state variable
  Integration : mylib/Integration  SystemSampleTime=-1  VariantActivationTime=update diagram  AllowFlexibleInterface=on  Latency=0  AutoFrameSizeCalculation=off
  Product : Product  Inputs=3
  Subtract : Sum  Inputs=+-
  "TCWR Inlet temperature of cooling water °C " : Subsystem
  TCWR-TWR : Sum  Inputs=+-
  "YY(37) " : Outport  VectorParamsAs1DForOutWhenUnconnected=off
  tag scope: TCWR=global, TWR=global
  wires:
  Divide2/1 -> Integration/1
  Initial state variable/1 -> Integration/2
  "TCWR Inlet temperature of cooling water °C "/1(TCWR) -> [TCWR], TCWR-TWR/1
  Integration/1 -> TCWR-TWR/2, "YY(37) "/1, [TWR]
  FWR/1 -> Product/1
  Constant6/1 -> Product/2
  TCWR-TWR/1 -> Product/3
  QUR/1 -> Divide1/1
  Constant1/1 -> Divide1/2
  Divide1/1 -> Divide/1
  Constant2/1 -> Divide/2
  Product/1 -> Subtract/1
  Divide/1 -> Subtract/2
  Subtract/1 -> Divide2/1
  HWR/1 -> Divide2/2
  Constant/1 -> Initial state variable/1

== system COSTEP_Exergy/Reactor/Reactor Heat exchanger/Reactor Heat exchanger/FWR Flow of cooling water to reactor gallons per minute ==
  VPOS(10) : Inport
  VRNG(10) : Inport  Port=2
  " " : Product  Inputs=**/
  Constant2 : Constant  Value=100
  FWR : Outport  VectorParamsAs1DForOutWhenUnconnected=off
  wires:
  Constant2/1 -> " "/3
  " "/1 -> FWR/1
  VPOS(10)/1 -> " "/1
  VRNG(10)/1 -> " "/2

== system COSTEP_Exergy/Reactor/Reactor Heat exchanger/Reactor Heat exchanger/Subsystem ==
  VLR : Inport
  Constant : Constant  Value=7.8
  Constant1 : Constant
  Constant2 : Constant  Value=0
  Constant3 : Constant  Value=0.025
  Constant4 : Constant  Value=0.25
  Divide : Product  Inputs=*/
  Divide1 : Product  Inputs=**
  If : If  IfExpression=u1 > 50  ElseIfExpressions=u1 < 10
  If Action Subsystem : Subsystem  TreatAsAtomicUnit=on
  If Action Subsystem1 : Subsystem  TreatAsAtomicUnit=on
  If Action Subsystem2 : Subsystem  TreatAsAtomicUnit=on
  Subtract : Sum  Inputs=+-
  UARLEV : Merge  Inputs=3
  "UARLEV " : Outport  VectorParamsAs1DForOutWhenUnconnected=off
  wires:
  If/2 -> If Action Subsystem1/Action
  If/1 -> If Action Subsystem/Action
  UARLEV/1 -> "UARLEV "/1
  If Action Subsystem1/1(Out1) -> UARLEV/2
  If Action Subsystem/1(Out1) -> UARLEV/1
  If/3 -> If Action Subsystem2/Action
  If Action Subsystem2/1(Out1) -> UARLEV/3
  VLR/1 -> Divide/1
  Constant/1 -> Divide/2
  Divide/1 -> Divide1/2, If/1
  Constant1/1 -> If Action Subsystem/1(In1)
  Constant2/1 -> If Action Subsystem1/1(In1)
  Constant3/1 -> Divide1/1
  Divide1/1 -> Subtract/1
  Constant4/1 -> Subtract/2
  Subtract/1 -> If Action Subsystem2/1(In1)

== system COSTEP_Exergy/Reactor/Reactor Heat exchanger/Reactor Heat exchanger/Subsystem2 ==
  UARLEV : Inport
  AGSP : Inport  Port=2
  Add : Sum  Inputs=++-
  Constant : Constant  Value=-0.5
  Constant1 : Constant  Value=2.75
  Constant2 : Constant  Value=2.5
  Constant3 : Constant  Value=855490E-6
  Math Function : Math  Operator=magnitude^2  SignedPower=on
  Product : Product
  Product1 : Product
  UAR : Product  Inputs=3
  "UAR " : Outport
  wires:
  Constant/1 -> Product/1
  Constant3/1 -> UAR/3
  AGSP/1 -> Product1/2, Math Function/1
  Add/1 -> UAR/2
  Product1/1 -> Add/2
  Math Function/1 -> Product/2
  Constant1/1 -> Product1/1
  Constant2/1 -> Add/3
  Product/1 -> Add/1
  UAR/1 -> "UAR "/1
  UARLEV/1 -> UAR/1
